simulink model "INS_GPS_sim"  (R2023b)
settings: Solver=ode4  StartTime=0.0  StopTime=418  FixedStep=0.01  RelTol=1e-3
InitFcn:
  | lin;
values from neighbouring files (symbols this model uses):
  A_num = A_func(x_num, u_num)    [init.m]    (also in lin.m)
  B_num = B_func(x_num, u_num)    [init.m]    (also in lin.m)
undefined symbols (not defined in the file or in its folder): Continuous, Time
libraries: ctrlSharedLib x1
settings Model: Creator=Ali  LastModifiedBy=Ali

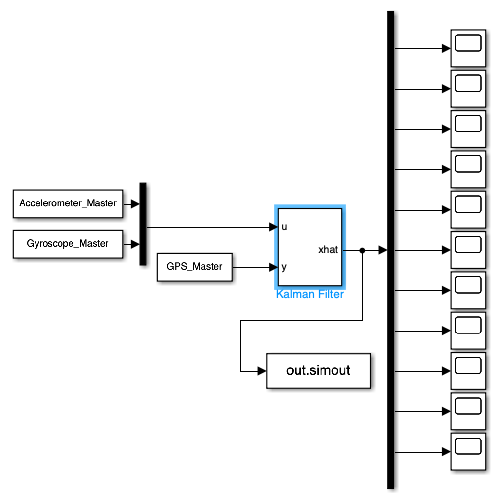
[thumbnail: Simulink's stored preview of the top-level diagram]
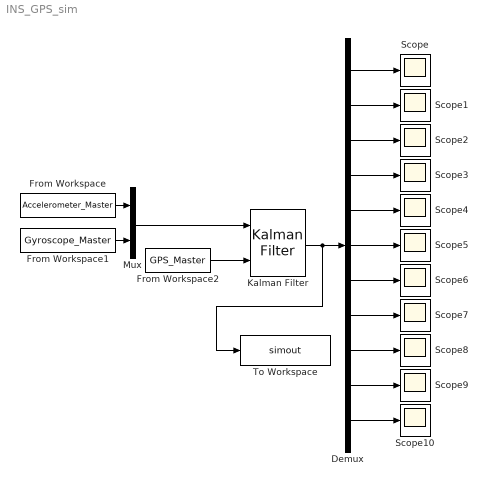
== system INS_GPS_sim ==
  Demux : Demux  Outputs=11
  From Workspace : FromWorkspace  VariableName=Accelerometer_Master
  From Workspace1 : FromWorkspace  VariableName=Gyroscope_Master
  From Workspace2 : FromWorkspace  VariableName=GPS_Master
  Kalman Filter : ctrlSharedLib/Kalman Filter  TimeDomain=Continuous-Time  UseCurrentEstimator=on  ModelSource=Individual A, B, C, D matrices  ModelSourceVariable=ss(0.95,1,1,0,1)  A=A_num  B=B_num  C=eye(6, 11)  D=0  NumberOfStates=1  NumberOfInputs=1  NumberOfOutputs=1  InitialEstimateSource=Dialog  X0=0  P0=10  UseK=off  UseGH=off  NumberOfProcessNoiseInputs=1  G=1  TimeInvariantG=on  H=0  TimeInvariantH=on  Q=50  TimeInvariantQ=on  R=100  TimeInvariantR=on  N=0  TimeInvariantN=on  AddInputPort=on  AddEnablePort=off  OutputEstimatedY=off  OutputP=off  Ts=-1
  Mux : Mux  Inputs=2
  Scope{,1..10} (11 alike) : Scope
  To Workspace : ToWorkspace  VariableName=simout  SaveFormat=Timeseries  SampleTime=-1
  wires:
  From Workspace/1 -> Mux/1
  From Workspace1/1 -> Mux/2
  Mux/1 -> Kalman Filter/1
  From Workspace2/1 -> Kalman Filter/2
  Kalman Filter/1 -> To Workspace/1, Demux/1
  Demux/1 -> Scope/1
  Demux/2 -> Scope1/1
  Demux/3 -> Scope2/1
  Demux/4 -> Scope3/1
  Demux/5 -> Scope4/1
  Demux/6 -> Scope5/1
  Demux/7 -> Scope6/1
  Demux/9 -> Scope8/1
  Demux/8 -> Scope7/1
  Demux/10 -> Scope9/1
  Demux/11 -> Scope10/1
